simulink model "sl_quadrotor_conference"  (R2018a)
settings: Solver=ode45  StartTime=0.0  StopTime=20  MaxStep=0.1  RelTol=1e-3  EnableMultiTasking=on
PreLoadFcn:
  | % load parameters of the default quadrotor
  | disp('Quadrotor parameters loaded by PreLoadFcn')
  | mdl_quadrotor
undefined symbols (not defined in the file or in its folder): quadrotor, rot2
libraries: roblocks x1, simulink x1
settings Model: Creator=corkep  LastModifiedBy=Henrik
settings DataIOCC: LimitDataPoints=on
settings OptimizationCC: ExpressionDepthLimit=2147483647  LifeSpan=inf
settings DebuggingCC: UnderspecifiedInitializationDetection=Classic  MergeDetectMultiDrivingBlocksExec=none  SolverPrmCheckMsg=warning  AllowSymbolicDim=off  StateNameClashWarn=warning  SFUnexpectedBacktrackingDiag=warning  SFNoUnconditionalDefaultTransitionDiag=warning  SFExecutionAtInitializationDiag=none
settings HardwareCC: ProdBitPerPointer=32  ProdBitPerSizeT=32  ProdBitPerPtrDiffT=32  ProdLargestAtomicFloat=None  ProdIntDivRoundTo=Undefined  ProdEndianess=Unspecified  ProdWordSize=32  ProdHWDeviceType=32-bit Generic
settings ModelReferenceCC: PropagateSignalLabelsOutOfModel=off
settings CodeAppCC: StateflowObjectComments=on
settings GRTTargetCC: TargetLangStandard=C89/C90 (ANSI)  GeneratePreprocessorConditionals=Disable all  CombineOutputUpdateFcns=off  GRTInterface=on
settings ConfigComp: CovMetricSettings=dw  CovHtmlReporting=on  CovSaveCumulativeToWorkspaceVar=on  CovSaveSingleToWorkspaceVar=on  CovExternalEMLEnable=off  CovSFcnEnable=off

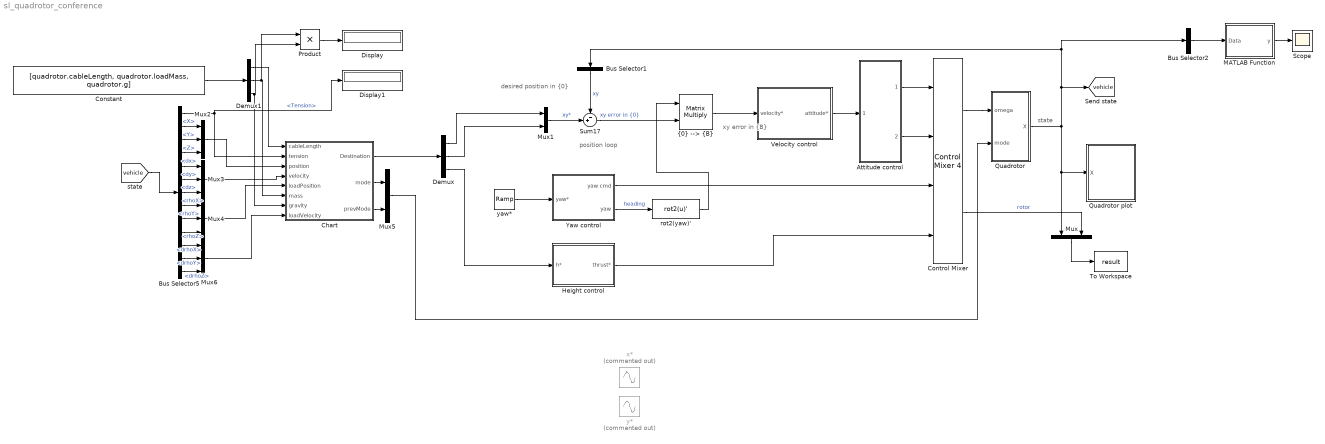
== system sl_quadrotor_conference ==
  note: xy error
      | in {B}
  note: desired position
      | in {0}
  note: position
      | loop
  note: state
  Attitude control : Subsystem  mask{P=100, D=1}
      mask prompts: P "Proportional gain"; D "Derivative gain"
  Bus Selector1 : BusSelector  OutputSignals=X,Y  OutputAsBus=on
  Bus Selector2 : BusSelector  OutputSignals=X,Y,rhoX,rhoY  OutputAsBus=on
  Bus Selector5 : BusSelector  OutputSignals=Tension,X,Y,Z,dx,dy,dz,rhoX,rhoY,rhoZ,drhoX,drhoY,drhoZ
  Chart : Stateflow chart  TreatAsAtomicUnit=on
  Constant : Constant  Value=[quadrotor.cableLength, quadrotor.loadMass, quadrotor.g]
  Control Mixer : roblocks/Vehicles/Control Mixer 4  quad=quadrotor  maxrot=1000  minrot=5
  Demux : Demux  Outputs=3
  Demux1 : Demux  Outputs=3
  Display : Display
  Display1 : Display
  Height control : Subsystem  mask{P=4, D=1, T0=40}
      mask prompts: P "Proportional gain"; D "Derivative gain"; T0 "Thrust feedforward"
  MATLAB Function : MATLAB Function  TreatAsAtomicUnit=on
  Mux : Mux  Inputs=2
  Mux1 : Mux  Inputs=2
  Mux{2..4,6} (4 alike) : Mux  Inputs=3
  Mux5 : Mux  Inputs=2
  Product : Product
  Quadrotor : Subsystem  AncestorBlock=roblocks/Vehicles/Quadrotor  mask{quad=quadrotor, x0=[0 1 -0.2], groundflag=on, mode=0}
      mask prompts: quad "Quadrotor params"; x0 "Initial position"; groundflag "Ground"
      mask help: Quadrotor dynamics
      mask Help:
      | Integrate spatial velocity to update pose represented as a homogeneous
      | transformation.
      | 
      | <b>Parameters::</b>
      | 
      | q (struct)  A structure containing quadrotor dynamics
      | 
      | The elements of q are:
      | 
      |  J         Flyer rotational inertia matrix (3x3)
      |  h         Height of rotors above CoG (1x1)
      |  d         Length of flyer arms (1x1)
      |  nb        Number of blades per rotor (1x1)
      |  r         Rotor radius (1x1)
      |  c         Blade chord (1x1)
      |  e         Flapping hinge offset (1x1)
      |  Mb        Rotor blade mass (1x1)
      |  Mc        Estimated hub clamp mass (1x1)
      |  ec        Blade root clamp displacement (1x1)
      |  Ib        Rotor blade rotational inertia (1x1)
      |  Ic        Estimated root clamp inertia (1x1)
      |  mb        Static blade moment (1x1)
      |  Ir        Total rotor inertia (1x1)
      |  Ct        Non-dim. thrust coefficient (1x1)
      |  Cq        Non-dim. torque coefficient (1x1)
      |  sigma     Rotor solidity ratio (1x1)
      |  thetat    Blade tip angle (1x1)
      |  theta0    Blade root angle (1x1)
      |  theta1    Blade twist angle (1x1)
      |  theta75   3/4 blade angle (1x1)
      |  thetai    Blade ideal root approximation (1x1)
      |  a         Lift slope gradient (1x1)
      |  A         Rotor disc area (1x1)
      |  gamma     Lock number (1x1)
      | 
      | 
      | <b>Inputs::</b>
      | 
      | w1 (1x1) angular velocity of rotor 1 [rad]
      | w2 (1x1) angular velocity of rotor 2 [rad]
      | w3 (1x1) angular velocity of rotor 3 [rad]
      | w4 (1x1) angular velocity of rotor 4 [rad]
      | 
      | <b>Outputs::</b>
      | 
      | X (1x12) state vector (x, y, z, thr, thp, thy, xd, yd, zd, thrd, thpd, thyd)
      | 
      | (x,y,z) is the position in the world frame [m]
      | (thr, thp, thy) the roll/pitch/yaw orientation in the world frame [rad]
      | (xd,yd,zd) is the velocity in the body frame [m]
      | (thrd,thpd,thyd) is the roll/pitch/yaw rates in the body frame [rad/s]
      | 
      | <b>Notes::</b>
      | 
      | - See also mdl_quadrotor which defines parameters for the ANU X4 flyer.
      mask Display:
      | port_label('input',1,'\varpi','texmode','on');
      | port_label('output',1,'X','texmode','on');
  Quadrotor plot : Subsystem  AncestorBlock=roblocks/Vehicles/Quadrotor plot  mask{quad=quadrotor, xydim=2, zdim=10}
      mask prompts: quad "Model"; xydim "xy-axes dimension"; zdim "z-axis dimension"
      mask help: Animate quadrotor.
      mask Help:
      | This block graphically displays a quadrotor (flying robot).
      | 
      | A new figure is created and A graphical model of a quadrotor is animated
      | to a pose specified by the state vector input to the block.
      | 
      | The state vector is [x y z roll pitch yaw] in world coordinates and the
      | angles are in radians.
      | 
      | Notes:
      | - The dimensions of the vehicle workspace are set by parameters
  Scope : Scope
  Sum17 : Sum  Inputs=-+|
  To Workspace : ToWorkspace  VariableName=result  SampleTime=-1
  Velocity control : Subsystem  mask{P=0.1, D=2}
      mask prompts: P "Proportional gain"; D "Derivative gain"
  Yaw control : Subsystem  mask{P=20, D=2}
      mask prompts: P "Proportional gain"; D "Derivative gain"
  rot2(yaw)' : MATLABFcn  MATLABFcn=rot2(u)'  OutputDimensions=[2 2]  Output1D=off
  x* : Sin  Commented=on  Frequency=2*pi*.125  Phase=-pi/2  SampleTime=0
  y* : Sin  Commented=on  Frequency=2*pi*.125  SampleTime=0
  yaw* : simulink/Sources/Ramp  slope=0.2  start=2  InitialOutput=0
  "{0} --> {B}" : Product  Multiplication=Matrix(*)  RndMeth=Zero
  tag scope: vehicle=global
  wires:
  Quadrotor/1(X) -> [vehicle], Bus Selector2/1, Bus Selector1/1, Quadrotor plot/1(X), Mux/1
  Mux/1 -> To Workspace/1
  Control Mixer/2 -> Mux/2  "rotor"
  Sum17/1 -> "{0} --> {B}"/2  "xy error in {0}"
  "{0} --> {B}"/1 -> Velocity control/1(velocity*)
  Velocity control/1(attitude*) -> Attitude control/1(attitude*)
  Yaw control/2(yaw) -> rot2(yaw)'/1  "heading"
  Yaw control/1(yaw cmd) -> Control Mixer/3
  yaw*/1 -> Yaw control/1(yaw*)
  Mux1/1 -> Sum17/2  "xy*"
  Bus Selector1/1 -> Sum17/1  "xy"
  rot2(yaw)'/1 -> "{0} --> {B}"/1
  Attitude control/1(roll torque*) -> Control Mixer/1
  Attitude control/2(pitch torque*) -> Control Mixer/2
  Control Mixer/1 -> Quadrotor/1(omega)
  Height control/1(thrust*) -> Control Mixer/4
  Bus Selector2/1 -> MATLAB Function/1(Data)
  MATLAB Function/1(y) -> Scope/1
  Chart/1(Destination) -> Demux/1
  Demux/1 -> Mux1/1
  Demux/2 -> Mux1/2
  Demux/3 -> Height control/1(h*)
  [vehicle] -> Bus Selector5/1
  Bus Selector5/1 -> Display1/1, Chart/2(tension)  "<Tension>"
  Bus Selector5/4 -> Mux2/3  "<Z>"
  Bus Selector5/2 -> Mux2/1  "<X>"
  Bus Selector5/3 -> Mux2/2  "<Y>"
  Bus Selector5/5 -> Mux3/1  "<dx>"
  Bus Selector5/6 -> Mux3/2  "<dy>"
  Bus Selector5/7 -> Mux3/3  "<dz>"
  Mux2/1 -> Chart/3(position)
  Mux3/1 -> Chart/4(velocity)
  Bus Selector5/8 -> Mux4/1  "<rhoX>"
  Bus Selector5/9 -> Mux4/2  "<rhoY>"
  Bus Selector5/10 -> Mux4/3  "<rhoZ>"
  Mux4/1 -> Chart/5(loadPosition)
  Constant/1 -> Demux1/1
  Demux1/1 -> Chart/1(cableLength)
  Demux1/2 -> Product/1, Chart/6(mass)
  Demux1/3 -> Product/2, Chart/7(gravity)
  Chart/2(mode) -> Mux5/1
  Chart/3(prevMode) -> Mux5/2
  Mux5/1 -> Quadrotor/2(mode)
  Bus Selector5/11 -> Mux6/1  "<drhoX>"
  Bus Selector5/12 -> Mux6/2  "<drhoY>"
  Bus Selector5/13 -> Mux6/3  "<drhoZ>"
  Mux6/1 -> Chart/8(loadVelocity)
  Product/1 -> Display/1

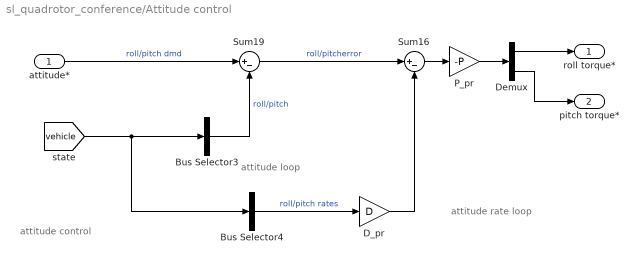
== system sl_quadrotor_conference/Attitude control ==
  note: attitude control
  note: attitude rate loop
  note: attitude loop
  attitude* : Inport
  Bus Selector3 : BusSelector  OutputSignals=roll,pitch  OutputAsBus=on
  Bus Selector4 : BusSelector  OutputSignals=droll,dpitch  OutputAsBus=on
  D_pr : Gain  Gain=D
  Demux : Demux  Outputs=2
  P_pr : Gain  Gain=-P
  Sum16 : Sum  Inputs=|+-
  Sum19 : Sum  Inputs=|+-
  roll torque* : Outport
  pitch torque* : Outport  Port=2
  wires:
  [vehicle] -> Bus Selector4/1, Bus Selector3/1
  attitude*/1 -> Sum19/1  "roll/pitch dmd"
  Bus Selector3/1 -> Sum19/2  "roll/pitch"
  Bus Selector4/1 -> D_pr/1  "roll/pitch rates"
  Sum19/1 -> Sum16/1  "roll/pitcherror"
  Sum16/1 -> P_pr/1
  P_pr/1 -> Demux/1
  D_pr/1 -> Sum16/2
  Demux/2 -> pitch torque*/1
  Demux/1 -> roll torque*/1

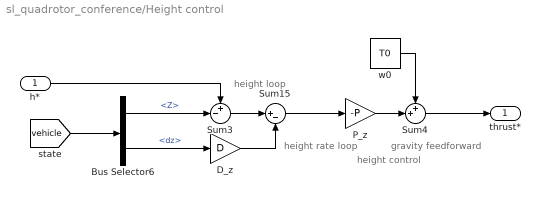
== system sl_quadrotor_conference/Height control ==
  note: height control
  note: gravity feedforward
  note: height rate
      | loop
  note: height
      | loop
  h* : Inport
  Bus Selector6 : BusSelector  OutputSignals=Z,dz
  D_z : Gain  Gain=D
  P_z : Gain  Gain=-P
  Sum15 : Sum  Inputs=|+-
  Sum3 : Sum  Inputs=+-|
  Sum4 : Sum  Inputs=++|
  w0 : Constant  Value=T0  SampleTime=0
  thrust* : Outport
  wires:
  w0/1 -> Sum4/1
  Sum15/1 -> P_z/1
  P_z/1 -> Sum4/2
  Bus Selector6/1 -> Sum3/2  "<Z>"
  h*/1 -> Sum3/1
  Sum3/1 -> Sum15/1
  Bus Selector6/2 -> D_z/1  "<dz>"
  D_z/1 -> Sum15/2
  Sum4/1 -> thrust*/1
  [vehicle] -> Bus Selector6/1

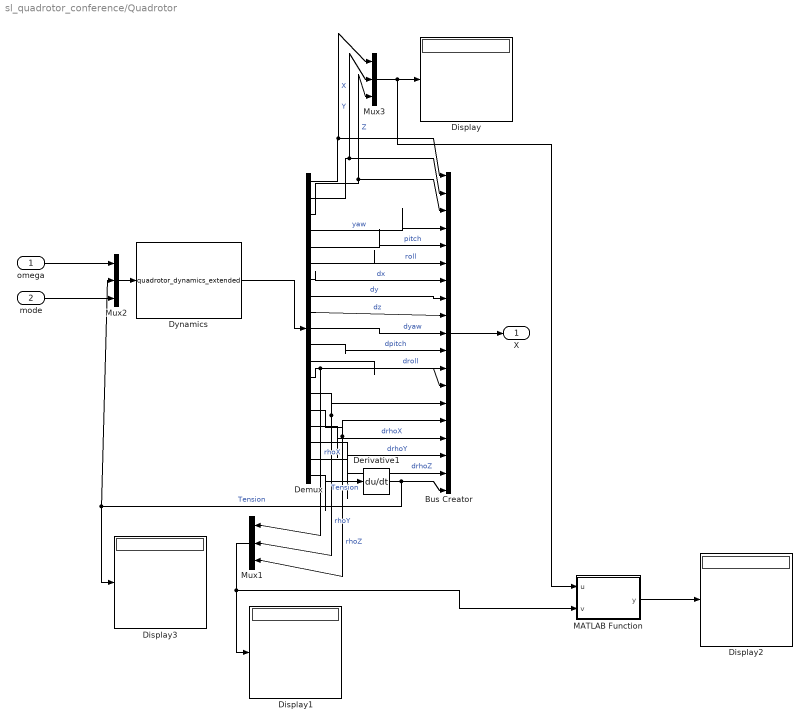
== system sl_quadrotor_conference/Quadrotor ==
  omega : Inport
  mode : Inport  Port=2
  Bus Creator : BusCreator  Inputs=19
  Demux : Demux  Outputs=19
  Derivative1 : Derivative
  Display{,1..3} (4 alike) : Display
  Dynamics : S-Function  FunctionName=quadrotor_dynamics_extended  Parameters=quad, x0, groundflag  SFunctionDeploymentMode=off  EnableBusSupport=off
  MATLAB Function : MATLAB Function  TreatAsAtomicUnit=on
  Mux1 : Mux  Inputs=3
  Mux2 : Mux  Inputs=3
  Mux3 : Mux  Inputs=3
  X : Outport
  wires:
  Demux/1 -> Mux3/1, Bus Creator/1  "X"
  Demux/3 -> Mux3/3, Bus Creator/3  "Z"
  Demux/4 -> Bus Creator/4  "yaw"
  Demux/5 -> Bus Creator/5  "pitch"
  omega/1 -> Mux2/1
  Demux/7 -> Bus Creator/7  "dx"
  Demux/9 -> Bus Creator/9  "dz"
  Demux/2 -> Mux3/2, Bus Creator/2  "Y"
  Demux/6 -> Bus Creator/6  "roll"
  Demux/8 -> Bus Creator/8  "dy"
  Bus Creator/1 -> X/1
  Dynamics/1 -> Demux/1
  Demux/10 -> Bus Creator/10  "dyaw"
  Demux/11 -> Bus Creator/11  "dpitch"
  Demux/12 -> Bus Creator/12  "droll"
  Mux1/1 -> MATLAB Function/2(v), Display1/1
  Demux/13 -> Mux1/1, Bus Creator/13  "rhoX"
  Demux/14 -> Bus Creator/14, Mux1/2  "rhoY"
  Demux/15 -> Mux1/3, Bus Creator/15  "rhoZ"
  Demux/16 -> Bus Creator/16  "drhoX"
  Demux/17 -> Bus Creator/17  "drhoY"
  Demux/18 -> Bus Creator/18  "drhoZ"
  Mux3/1 -> MATLAB Function/1(u), Display/1
  MATLAB Function/1(y) -> Display2/1
  Demux/19 -> Derivative1/1  "Tension"
  Mux2/1 -> Dynamics/1
  Derivative1/1 -> Display3/1, Mux2/2, Bus Creator/19  "Tension"
  mode/1 -> Mux2/3

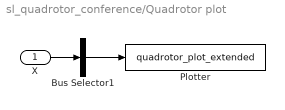
== system sl_quadrotor_conference/Quadrotor plot ==
  X : Inport
  Bus Selector1 : BusSelector  OutputSignals=X,Y,Z,yaw,pitch,roll,rhoX,rhoY,rhoZ  OutputAsBus=on
  Plotter : S-Function  FunctionName=quadrotor_plot_extended  Parameters=[xydim, zdim], 1, 1,quad  SFunctionDeploymentMode=off  EnableBusSupport=off
  wires:
  X/1 -> Bus Selector1/1
  Bus Selector1/1 -> Plotter/1

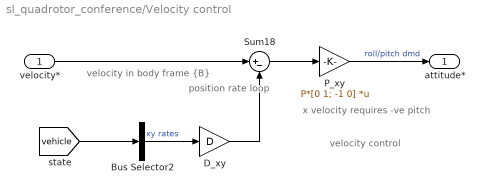
== system sl_quadrotor_conference/Velocity control ==
  note: x velocity requires -ve pitch
  note: velocity in body frame {B}
  note: velocity control
  note: position rate
      | loop
  velocity* : Inport
  Bus Selector2 : BusSelector  OutputSignals=dx,dy  OutputAsBus=on
  D_xy : Gain  Gain=D
  P_xy : Gain  Gain=P*[0 1; -1 0]  Multiplication=Matrix(K*u)
  Sum18 : Sum  Inputs=|+-
  attitude* : Outport
  wires:
  Bus Selector2/1 -> D_xy/1  "xy rates"
  D_xy/1 -> Sum18/2
  Sum18/1 -> P_xy/1
  velocity*/1 -> Sum18/1
  [vehicle] -> Bus Selector2/1
  P_xy/1 -> attitude*/1  "roll/pitch dmd"

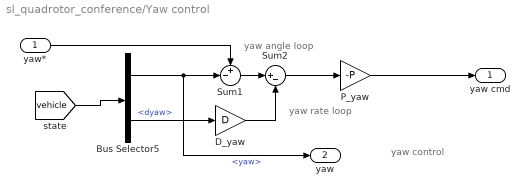
== system sl_quadrotor_conference/Yaw control ==
  note: yaw control
  note: yaw rate
      | loop
  note: yaw angle
      | loop
  yaw* : Inport
  Bus Selector5 : BusSelector  OutputSignals=yaw,dyaw
  D_yaw : Gain  Gain=D
  P_yaw : Gain  Gain=-P
  Sum1 : Sum  Inputs=+-|
  Sum2 : Sum  Inputs=|+-
  yaw cmd : Outport
  yaw : Outport  Port=2
  wires:
  [vehicle] -> Bus Selector5/1
  P_yaw/1 -> yaw cmd/1
  Bus Selector5/1 -> yaw/1, Sum1/2  "<yaw>"
  Sum2/1 -> P_yaw/1
  Bus Selector5/2 -> D_yaw/1  "<dyaw>"
  D_yaw/1 -> Sum2/2
  Sum1/1 -> Sum2/1
  yaw*/1 -> Sum1/1

== matlab function sl_quadrotor_conference/MATLAB Function ==
  data: Data input; y output
function y = fcn(Data)

u = [Data(1); Data(2)];  
v = [Data(3); Data(4)];  

y = norm(u-v);

== matlab function sl_quadrotor_conference/Quadrotor/MATLAB Function ==
  data: u input; y output; v input
function y = fcn(u,v)

y = norm(u-v);

== stateflow chart sl_quadrotor_conference/Chart ==
  state Init
    during:
    Destination = [0; 0; -cableLength/2];
    mode = 0;
    prevMode = 0;
  state MoveSetup
    exit:
    Destination = [0; 0; -cableLength];
  state Setup
    entry: mode = 0;
    exit: prevMode = 0;
  state MovePull
    exit:
    Destination = [0; 0; -cableLength-0.1];
  state Pull
    entry: mode = 1;
    exit: prevMode = 1;
  state MoveRaise
    exit:
    Destination = [0; 0; -cableLength*3];
  state Raise
    entry: mode = 2;
    exit: prevMode = 2;
  (default) -> Init
  Init -> MoveSetup : [norm(velocity) < 0.05 && norm(Destination-position) < 0.2]
  MoveSetup -> Setup
  Pull -> Setup [order 2] : [norm(position-loadPosition)<cableLength]
  Setup -> MovePull : [norm(position-loadPosition)>=cableLength]
  MovePull -> Pull
  Raise -> Pull : [norm(position-loadPosition)<=cableLength]
  Pull -> MoveRaise [order 1] : [tension > mass*gravity && norm(position-loadPosition)>=cableLength]
  MoveRaise -> Raise
  data: cableLength input size=1; tension input size=1; position input size=3; velocity input size=3; Destination output size=3; loadPosition input size=3; mass input size=1; gravity input size=1; mode output size=1; prevMode output size=1; loadVelocity input size=3
